simulink model "Prediction_Horizon_Generator"  (R2016b)
settings: Solver=FixedStepDiscrete  StartTime=0.0  StopTime=inf  FixedStep=PredtnHrznGenr.tiSimnTiStep_C  RelTol=1e-3  EnableMultiTasking=on
settings Model: Creator=djuenema  LastModifiedBy=djuenema
settings DataIOCC: SaveFormat=StructureWithTime  SaveOutput=off  DSMLogging=off  VisualizeSimOutput=off  SaveTime=off  SignalLoggingName=Results
settings OptimizationCC: BlockReduction=off  ConditionallyExecuteInputs=off  LifeSpan=inf
settings DebuggingCC: AllowSymbolicDim=off  SFUnexpectedBacktrackingDiag=warning  SFNoUnconditionalDefaultTransitionDiag=warning  SFExecutionAtInitializationDiag=none
settings ModelReferenceCC: ModelReferenceNumInstancesAllowed=Single  PropagateSignalLabelsOutOfModel=off
settings GRTTargetCC: TargetLangStandard=C89/C90 (ANSI)
settings ConfigComp: CovMetricSettings=dw  CovHtmlReporting=on  CovSaveCumulativeToWorkspaceVar=on  CovSaveSingleToWorkspaceVar=on  CovExternalEMLEnable=off

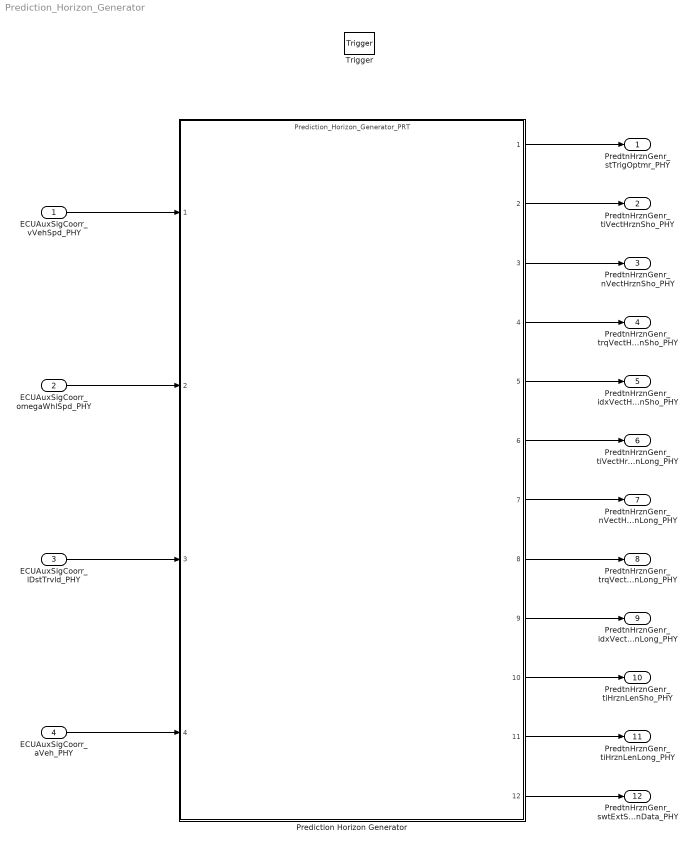
== system Prediction_Horizon_Generator ==
  ECUAuxSigCoorr_vVehSpd_PHY : Inport
  ECUAuxSigCoorr_omegaWhlSpd_PHY : Inport  Port=2
  ECUAuxSigCoorr_lDstTrvld_PHY : Inport  Port=3
  ECUAuxSigCoorr_aVeh_PHY : Inport  Port=4
  Trigger : TriggerPort  TriggerType=function-call  VariantControl=Variant  PortDimensions=1
  Prediction Horizon Generator : ModelReference  ModelNameDialog=Prediction_Horizon_Generator_PRT.slxp  ModelReferenceVersion=1.3  CopyOfModelProtected=on
  PredtnHrznGenr_stTrigOptmr_PHY : Outport
  PredtnHrznGenr_tiVectHrznSho_PHY : Outport  Port=2
  PredtnHrznGenr_nVectHrznSho_PHY : Outport  Port=3
  PredtnHrznGenr_trqVectHrznSho_PHY : Outport  Port=4
  PredtnHrznGenr_idxVectHrznLenSho_PHY : Outport  Port=5
  PredtnHrznGenr_tiVectHrznLong_PHY : Outport  Port=6
  PredtnHrznGenr_nVectHrznLong_PHY : Outport  Port=7
  PredtnHrznGenr_trqVectHrznLong_PHY : Outport  Port=8
  PredtnHrznGenr_idxVectHrznLenLong_PHY : Outport  Port=9
  PredtnHrznGenr_tiHrznLenSho_PHY : Outport  Port=10
  PredtnHrznGenr_tiHrznLenLong_PHY : Outport  Port=11
  PredtnHrznGenr_swtExtSrcPredtnData_PHY : Outport  Port=12
  wires:
  ECUAuxSigCoorr_vVehSpd_PHY/1 -> Prediction Horizon Generator/1
  ECUAuxSigCoorr_lDstTrvld_PHY/1 -> Prediction Horizon Generator/3
  ECUAuxSigCoorr_omegaWhlSpd_PHY/1 -> Prediction Horizon Generator/2
  ECUAuxSigCoorr_aVeh_PHY/1 -> Prediction Horizon Generator/4
  Prediction Horizon Generator/8 -> PredtnHrznGenr_trqVectHrznLong_PHY/1
  Prediction Horizon Generator/9 -> PredtnHrznGenr_idxVectHrznLenLong_PHY/1
  Prediction Horizon Generator/10 -> PredtnHrznGenr_tiHrznLenSho_PHY/1
  Prediction Horizon Generator/11 -> PredtnHrznGenr_tiHrznLenLong_PHY/1
  Prediction Horizon Generator/12 -> PredtnHrznGenr_swtExtSrcPredtnData_PHY/1
  Prediction Horizon Generator/1 -> PredtnHrznGenr_stTrigOptmr_PHY/1
  Prediction Horizon Generator/3 -> PredtnHrznGenr_nVectHrznSho_PHY/1
  Prediction Horizon Generator/4 -> PredtnHrznGenr_trqVectHrznSho_PHY/1
  Prediction Horizon Generator/5 -> PredtnHrznGenr_idxVectHrznLenSho_PHY/1
  Prediction Horizon Generator/2 -> PredtnHrznGenr_tiVectHrznSho_PHY/1
  Prediction Horizon Generator/6 -> PredtnHrznGenr_tiVectHrznLong_PHY/1
  Prediction Horizon Generator/7 -> PredtnHrznGenr_nVectHrznLong_PHY/1
